simulink model "PickAndPlace_Simulation_QLabs"  (R2024b)
settings: Solver=FixedStepDiscrete  StartTime=0.0  StopTime=inf  FixedStep=0.005  RelTol=1e-3
InitFcn:
  | qarmRigidBodyTree = importrobot('Resources/qarm/urdf/QARM.urdf');
  | qarmRigidBodyTree.Bodies{1,3}.Joint.PositionLimits(1) = -pi/4;
  | show(qarmRigidBodyTree);
undefined symbols (not defined in the file or in its folder): EFFECTOR, END, HIL, Levenberg, Marquardt, qc_get_step_size
libraries: quarc_library x5, robotmaniplib x2
settings Model: Creator=MLevis  LastModifiedBy=tedzh
settings DebuggingCC: UnconnectedInputMsg=warning  UnconnectedOutputMsg=warning  UnconnectedLineMsg=warning
settings ModelReferenceCC: EnableRefExpFcnMdlSchedulingChecks=on
settings RTWCC: GenCodeOnly=on  GPUComputeCapability=3.5  DLArmComputeVersion=19.05

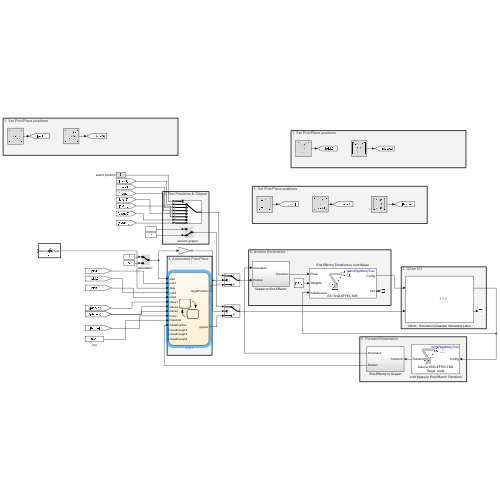
[thumbnail: Simulink's stored preview of the top-level diagram]
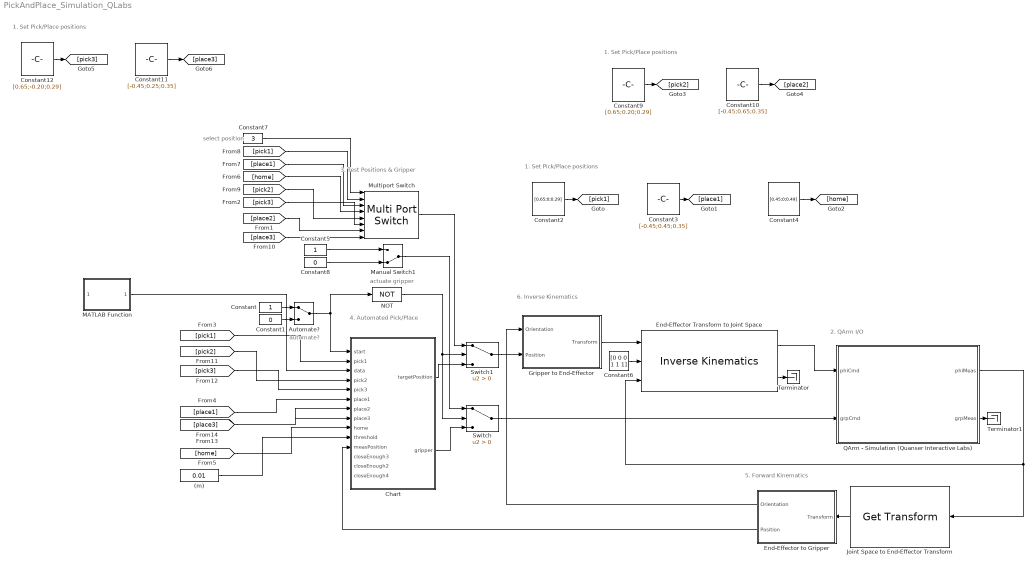
== system PickAndPlace_Simulation_QLabs ==
  note: 6. Inverse Kinematics
  note: 1. Set Pick/Place positions
  note: 4. Automated Pick/Place
  note: 2. QArm I/O
  note: 3. Test Positions & Gripper
  note: select position
  note: actuate gripper
  note: 5. Forward Kinematics
  note: automate?
  note: 1. Set Pick/Place positions
  note: 1. Set Pick/Place positions
  (m) : Constant  Value=0.01
  Automate? : ManualSwitch
  Chart : Stateflow chart  TreatAsAtomicUnit=on
  Constant : Constant
  Constant1 : Constant  Value=0
  Constant10 : Constant  Value=[-0.45;0.65;0.35]  VectorParams1D=off
  Constant11 : Constant  Value=[-0.45;0.25;0.35]  VectorParams1D=off
  Constant12 : Constant  Value=[0.65;-0.20;0.29]  VectorParams1D=off
  Constant2 : Constant  Value=[0.65;0;0.29]  VectorParams1D=off
  Constant3 : Constant  Value=[-0.45;0.45;0.35]  VectorParams1D=off
  Constant4 : Constant  Value=[0.45;0;0.49]  VectorParams1D=off
  Constant5 : Constant
  Constant6 : Constant  Value=[0 0 0 1 1 1]
  Constant7 : Constant  Value=3
  Constant8 : Constant  Value=0
  Constant9 : Constant  Value=[0.65;0.20;0.29]  VectorParams1D=off
  End-Effector Transform to Joint Space : robotmaniplib/Inverse Kinematics  RigidBodyTree=qarmRigidBodyTree  EndEffector=END-EFFECTOR  ShowInfo=on  SolverName=Levenberg-Marquardt  EnforceJointLimits=on  MaxIterations=2  MaxTime=qc_get_step_size  GradientTolerance=1e-4  SolutionTolerance=1e-3  StepTolerance=1e-3  ErrorChangeTolerance=1e-6  UseErrorDamping=on  DampingBias=0.0025  SimulateUsing=Code generation
  End-Effector to Gripper : Subsystem
  Gripper to End-Effector : Subsystem
  Joint Space to End-Effector Transform : robotmaniplib/Get Transform  RigidBodyTree=qarmRigidBodyTree  SourceBody=END-EFFECTOR  TargetBody=world  SimulateUsing=Interpreted execution
  MATLAB Function : MATLAB Function  TreatAsAtomicUnit=on
  Manual Switch1 : ManualSwitch  CurrentSetting=0
  Multiport Switch : MultiPortSwitch  Inputs=7  SaturateOnIntegerOverflow=off  InputSameDT=off
  NOT : Logic  Operator=NOT  IconShape=distinctive  AllPortsSameDT=off  OutDataTypeStr=boolean
  QArm - Simulation (Quanser Interactive Labs) : Subsystem
      mask Display:
      | image('Resources/QArm.png')
      | port_label('input', 1, 'phiCmd');
      | port_label('input', 2, 'grpCmd');
      | port_label('output', 1, 'phiMeas');
      | port_label('output', 2, 'grpMeas');
  Switch : Switch  Criteria=u2 > Threshold  SaturateOnIntegerOverflow=off  InputSameDT=off
  Switch1 : Switch  Criteria=u2 > Threshold  SaturateOnIntegerOverflow=off  InputSameDT=off
  Terminator : Terminator
  Terminator1 : Terminator
  wires:
  End-Effector to Gripper/1(Orientation) -> Gripper to End-Effector/1(Orientation)
  Constant4/1 -> [home]
  [place1] -> Multiport Switch/3
  Manual Switch1/1 -> Switch/1
  NOT/1 -> Switch1/2, Switch/2
  [home] -> Chart/9(home)
  QArm - Simulation (Quanser Interactive Labs)/1(phiMeas) -> End-Effector Transform to Joint Space/3, Joint Space to End-Effector Transform/1
  End-Effector Transform to Joint Space/2 -> Terminator/1
  Switch/1 -> QArm - Simulation (Quanser Interactive Labs)/2(grpCmd)
  [place1] -> Chart/6(place1)
  (m)/1 -> Chart/10(threshold)
  [pick1] -> Chart/2(pick1)
  Constant/1 -> Automate?/1
  Joint Space to End-Effector Transform/1 -> End-Effector to Gripper/1(Transform)
  Constant3/1 -> [place1]
  QArm - Simulation (Quanser Interactive Labs)/2(grpMeas) -> Terminator1/1
  End-Effector to Gripper/2(Position) -> Chart/11(measPosition)
  End-Effector Transform to Joint Space/1 -> QArm - Simulation (Quanser Interactive Labs)/1(phiCmd)
  Constant8/1 -> Manual Switch1/2
  Automate?/1 -> NOT/1, Chart/1(start)
  Switch1/1 -> Gripper to End-Effector/2(Position)
  Constant6/1 -> End-Effector Transform to Joint Space/2
  Constant7/1 -> Multiport Switch/1
  Multiport Switch/1 -> Switch1/1
  Chart/1(targetPosition) -> Switch1/3
  Constant5/1 -> Manual Switch1/1
  Chart/2(gripper) -> Switch/3
  [pick1] -> Multiport Switch/2
  [home] -> Multiport Switch/4
  Gripper to End-Effector/1(Transform) -> End-Effector Transform to Joint Space/1
  Constant2/1 -> [pick1]
  Constant1/1 -> Automate?/2
  Constant9/1 -> [pick2]
  Constant10/1 -> [place2]
  Constant11/1 -> [place3]
  Constant12/1 -> [pick3]
  [pick2] -> Multiport Switch/5
  [pick3] -> Multiport Switch/6
  [place2] -> Multiport Switch/7
  [place3] -> Multiport Switch/8
  [pick2] -> Chart/4(pick2)
  [pick3] -> Chart/5(pick3)
  [place2] -> Chart/7(place2)
  [place3] -> Chart/8(place3)
  MATLAB Function/1(fruitType) -> Chart/3(data)

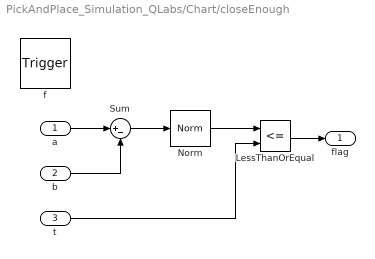
== system PickAndPlace_Simulation_QLabs/Chart/closeEnough ==
  a : Inport  OutDataTypeStr=double  PortDimensions=[3,1]
  b : Inport  Port=2  OutDataTypeStr=double  PortDimensions=[3,1]
  t : Inport  Port=3  OutDataTypeStr=double  PortDimensions=[1]
  f : TriggerPort  TriggerType=function-call  VariantControl=(inherit)
      settings: CopyFcn=Stateflow.SLINSF.SimulinkMan.removeBlockPreDeleteFcn  PreDeleteFcn=Stateflow.SLINSF.SimulinkMan.unsafePredeleteFcn
  LessThanOrEqual : RelationalOperator  Operator=<=  OutDataTypeStr=boolean  RndMeth=Simplest  InputSameDT=off
  Norm : quarc_library/Math Operations/Vectors/Norm
      settings: SourceProductName=QUARC Targets
  Sum : Sum  Inputs=|+-
  flag : Outport  VectorParamsAs1DForOutWhenUnconnected=off
  wires:
  a/1 -> Sum/1
  b/1 -> Sum/2
  Sum/1 -> Norm/1
  Norm/1 -> LessThanOrEqual/1
  t/1 -> LessThanOrEqual/2
  LessThanOrEqual/1 -> flag/1

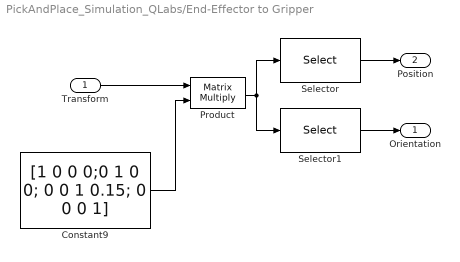
== system PickAndPlace_Simulation_QLabs/End-Effector to Gripper ==
  Transform : Inport
  Constant9 : Constant  Value=[1 0 0 0;0 1 0 0; 0 0 1 0.15; 0 0 0 1]  VectorParams1D=off
  Product : Product  Multiplication=Matrix(*)
  Selector : Selector  NumberOfDimensions=2  InputPortWidth=3  IndexOptions=Index vector (dialog),Index vector (dialog)  Indices=[1:3],4  OutputSizes=1,1
  Selector1 : Selector  NumberOfDimensions=2  InputPortWidth=3  IndexOptions=Index vector (dialog),Index vector (dialog)  Indices=[1:3],[1:3]  OutputSizes=1,1
  Orientation : Outport
  Position : Outport  Port=2
  wires:
  Transform/1 -> Product/1
  Product/1 -> Selector/1, Selector1/1
  Selector/1 -> Position/1
  Constant9/1 -> Product/2
  Selector1/1 -> Orientation/1

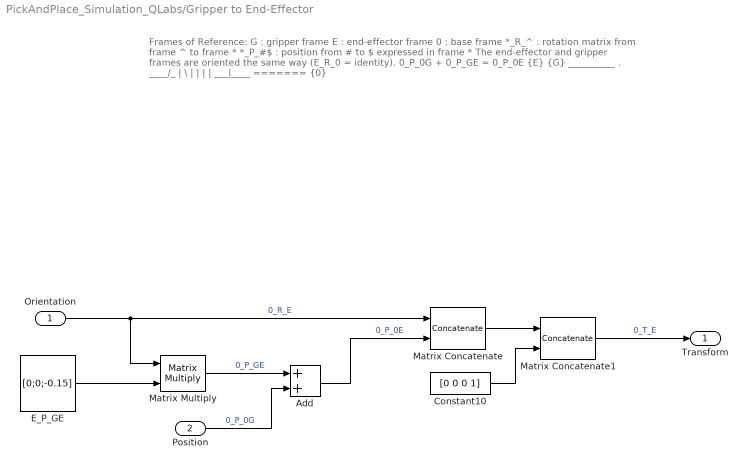
== system PickAndPlace_Simulation_QLabs/Gripper to End-Effector ==
  note: Frames of Reference:
      |
      | G : gripper frame
      | E : end-effector frame
      | 0 : base frame
      | *_R_^ : rotation matrix from frame ^ to frame *
      | *_P_#$ : position from # to $ expressed in frame *
      |
      | The end-effector and gripper frames are oriented the same way (E_R_0 = identity).
      | 0_P_0G + 0_P_GE = 0_P_0E
      |
      | {E} {G}
      | __________ . ____/_
      | | \
      | |
      | |
      | |
      | |
      | ___|____
      | =======
      | {0}
  Orientation : Inport
  Position : Inport  Port=2
  Add : Sum
  Constant10 : Constant  Value=[0 0 0 1]  VectorParams1D=off
  E_P_GE : Constant  Value=[0;0;-0.15]  VectorParams1D=off
  Matrix Concatenate : Concatenate  Mode=Multidimensional array  ConcatenateDimension=2
  Matrix Concatenate1 : Concatenate  Mode=Multidimensional array
  Matrix Multiply : Product  Multiplication=Matrix(*)
  Transform : Outport
  wires:
  Matrix Concatenate/1 -> Matrix Concatenate1/1
  Orientation/1 -> Matrix Concatenate/1, Matrix Multiply/1  "0_R_E"
  Constant10/1 -> Matrix Concatenate1/2
  Matrix Concatenate1/1 -> Transform/1  "0_T_E"
  Matrix Multiply/1 -> Add/1  "0_P_GE"
  Position/1 -> Add/2  "0_P_0G"
  E_P_GE/1 -> Matrix Multiply/2
  Add/1 -> Matrix Concatenate/2  "0_P_0E"

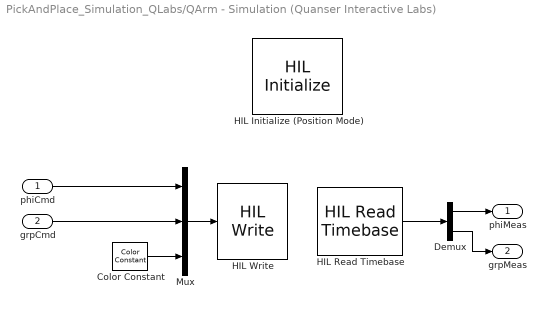
== system PickAndPlace_Simulation_QLabs/QArm - Simulation (Quanser Interactive Labs) ==
  phiCmd : Inport
  grpCmd : Inport  Port=2
  Color Constant : quarc_library/Sources/Signals/Color Constant  color=[0 1 0]
      settings: SourceProductName=QUARC Targets
  Demux : Demux  Outputs=[4 1]
  HIL Initialize (Position Mode) : quarc_library/Data Acquisition/Generic/Configuration/HIL Initialize  object_name=HIL-1  board_type=qarm_usb  board_number=0@tcpip://localhost:18900?nagle='off'  board_options=j0_mode=0;j1_mode=0;j2_mode=0;j3_mode=0;gripper_mode=0;  exclusive=off  active=on  hardware_clocks=[0]  clock_modes=[]  initial_clock_frequencies=[]  set_clock_params_at_start=off  set_clock_params_at_switch_in=off  set_clock_frequencies_at_start=off  set_clock_frequencies_at_switch_in=off  analog_input_channels=[5:9]  analog_input_configurations=[]  analog_input_maximums=[]  analog_input_minimums=[]  set_analog_input_params_at_start=off  set_analog_input_params_at_switch_in=off  analog_output_channels=[]  analog_output_maximums=inf  analog_output_minimums=-inf  initial_analog_outputs=[0]  final_analog_outputs=[0]  watchdog_analog_outputs=[]  set_analog_output_params_at_start=off  set_analog_output_params_at_switch_in=off  set_analog_outputs_at_start=off  set_analog_outputs_at_switch_in=off  set_analog_outputs_at_terminate=off  set_analog_outputs_at_switch_out=off  set_analog_outputs_on_watchdog=off  digital_input_channels=[]  digital_output_channels=[]  digital_output_configuration=[]  initial_digital_outputs=[0]  final_digital_outputs=[0]  watchdog_digital_outputs=[0]  set_digital_output_params_at_start=off  set_digital_output_params_at_switch_in=off  set_digital_outputs_at_start=off  set_digital_outputs_at_switch_in=off  set_digital_outputs_at_terminate=off  set_digital_outputs_at_switch_out=off  set_digital_outputs_on_watchdog=off  encoder_channels=[]  quadrature=[]  encoder_filter_frequency=[]  initial_encoder_counts=[]  set_encoder_params_at_start=off  set_encoder_params_at_switch_in=off  set_encoder_counts_at_start=off  set_encoder_counts_at_switch_in=off  pwm_channels=[]  pwm_modes=[]  pwm_frequency=[]  pwm_configuration=[]  pwm_alignment=[]  pwm_polarity=[]  pwm_leading_deadband=[]  pwm_trailing_deadband=[]  initial_pwm_outputs=[]  final_pwm_outputs=[]  watchdog_pwm_outputs=[]  set_pwm_params_at_start=off  set_pwm_params_at_switch_in=off  set_pwm_outputs_at_start=off  set_pwm_outputs_at_switch_in=off  set_pwm_outputs_at_terminate=off  set_pwm_outputs_at_switch_out=off  set_pwm_outputs_on_watchdog=off  other_output_channels=[1000:1004 11000:11003 11005:11007]  initial_other_outputs=[zeros(1,9), ones(1,3)]  final_other_outputs=[zeros(1,9), ones(1,3)]  watchdog_other_outputs=zeros(1,12)  set_other_outputs_at_start=off  set_other_outputs_at_switch_in=off  set_other_outputs_at_terminate=on  set_other_outputs_at_switch_out=off  set_other_outputs_on_watchdog=off
      settings: AttributesFormatString=%<object_name> (%<board_type>-%<board_number>)
  HIL Read Timebase : quarc_library/Data Acquisition/Generic/Timebases/HIL Read Timebase  object_name=HIL-1  clock=0  analog_channels=[]  encoder_channels=[]  digital_channels=[]  other_channels=[1000:1004]  active=on  vector_output=on  data_type_mode=Inherit via back propagation  encoder_data_type=double  digital_data_type=boolean  overflow_mode=Synchronize (for simulated cards only)  samples_in_buffer=max(ceil(1/qc_get_step_size), 1)
  HIL Write : quarc_library/Data Acquisition/Generic/Immediate I//O/HIL Write  object_name=HIL-1  analog_channels=[]  pwm_channels=[]  digital_channels=[]  other_channels=[1000:1004 11005:11007]  sample_time=-1  active=on  vector_input=on
  Mux : Mux  Inputs=3
  phiMeas : Outport
  grpMeas : Outport  Port=2
  wires:
  Mux/1 -> HIL Write/1
  grpCmd/1 -> Mux/2
  Color Constant/1 -> Mux/3
  HIL Read Timebase/1 -> Demux/1
  phiCmd/1 -> Mux/1
  Demux/1 -> phiMeas/1
  Demux/2 -> grpMeas/1

== matlab function PickAndPlace_Simulation_QLabs/MATLAB Function ==
  data: dummy input; fruitType output int32
function fruitType = fcn(dummy)

coder.extrinsic('py.yolo_simulink.detect_fruit');

fruitType = int32(0);

result = py.yolo_simulink.detect_fruit(dummy);

fruitType = int32(result);

end

== stateflow chart PickAndPlace_Simulation_QLabs/Chart ==
  state Wait1
    gripper=0;
    targetPosition=home;
  state Detect1
    detectedType = data;
  state GotoPick1
    targetPosition=pick1;
    flag = closeEnough(measPosition, targetPosition, threshold);
  state CloseGripper1
    gripper=1;
  state GotoHome1
    targetPosition=home;
    flag = closeEnough(measPosition, targetPosition, threshold);
  state OpenGripper1
    gripper=0;
  state GotoPlace1
    fprintf('[Detect1] detectedType = %d\n', detectedType);
    switch detectedType
    case 1
    targetPosition = place1;  % strawberry
    case 2
    targetPosition = place2;  % banana
    case 3
    targetPosition = place3;  % tomato
    end
    flag = closeEnough(measPosition, targetPosition, threshold);
  state Wait [commented out]
    gripper=0;
    index = 0;
    targetPosition=home;
  state flag = closeEnough(a,b,t) [function]
  state GotoPick [commented out]
    switch mod(index,3)
    case 0
    targetPosition = pick1;
    case 1
    targetPosition = pick2;
    case 2
    targetPosition = pick3;
    end
    flag = closeEnough(measPosition, targetPosition, threshold);
  state CloseGripper [commented out]
    gripper=1;
  state GotoHome [commented out]
    targetPosition=home;
    flag = closeEnough(measPosition, targetPosition, threshold);
  state GotoPlace [commented out]
    targetPosition=place1;
    flag = closeEnough(measPosition, targetPosition, threshold);
  state OpenGripper [commented out]
    gripper=0;
    index = index+1;
  (default) -> Wait1
  GotoPick1 -> Detect1 : [after(2,sec) && flag]
  Wait1 -> GotoPick1 : [start && after(2,sec)]
  Detect1 -> CloseGripper1 : [after(5,sec) && detectedType > 0]
  GotoHome1 -> GotoPick1 [order 2] : [after(2,sec) && flag]
  CloseGripper1 -> GotoHome1 : [after(2,sec)]
  GotoHome1 -> GotoPlace1 [order 1] : [gripper && after(2,sec) && flag]
  OpenGripper1 -> GotoHome1 : [after(2,sec)]
  GotoPlace1 -> OpenGripper1 : [after(3,sec) && flag]
  (default) -> Wait [commented out]
  Wait -> GotoPick [commented out] : [start && after(2,sec)]
  GotoPick -> CloseGripper [commented out] : [after(2,sec)]
  CloseGripper -> GotoHome [commented out] : [after(2,sec)]
  GotoHome -> GotoPick [commented out] : [after(2,sec) ]
  GotoHome -> GotoPlace [commented out] : [gripper && after(2,sec)]
  OpenGripper -> GotoHome [commented out] : [after(2,sec)]
  GotoPlace -> OpenGripper [commented out] : [after(3,sec) && flag]
  data: a function_input double size=[3,1]; b function_input double size=[3,1]; flag function_output; t function_input double size=[1]; start input; pick1 input size=[3,1]; data input; pick2 input; pick3 input; targetPosition output size=[3,1]; gripper output size=[1]; place1 input double size=[3,1]; place2 input; place3 input; home input double size=[3,1]; threshold input; measPosition input double size=[3,1]; flag local; index local; detectedType local; closeEnough3 input; closeEnough2 input; closeEnough4 input double
